simulink model "Disturbance_Rejection"  (R2025b)
settings: Solver=VariableStepAuto  StartTime=0.0  StopTime=t_sim  RelTol=1e-5  EnableMultiTasking=on
values from neighbouring files (symbols this model uses):
  Am = [0 1; -wn_model^2 -2*zeta_model*wn_model]    [MRC_DistReject.m]    (also in MRC_Simulation.m; MRC_Simulation1.m; MRC_Simulation2.m)
  Ap = [0   1;  -wn^2   -2*zeta*wn]    [MRC_DistReject.m]    (also in MRC_Simulation.m; MRC_Simulation1.m; MRC_Simulation2.m)
  Bm = [0; 1]    [MRC_DistReject.m]    (also in MRC_Simulation.m; MRC_Simulation1.m; MRC_Simulation2.m)
  Bp = [0;  1]    [MRC_DistReject.m]    (also in MRC_Simulation.m; MRC_Simulation1.m; MRC_Simulation2.m)
  Cm = eye(2)    [MRC_DistReject.m]    (also in MRC_Simulation.m; MRC_Simulation1.m; MRC_Simulation2.m)
  Dm = [0;0]    [MRC_DistReject.m]    (also in MRC_Simulation.m; MRC_Simulation1.m; MRC_Simulation2.m)
  step1 = 0    [MRC_DistReject.m]    (also in MRC_Simulation.m = 0.2; MRC_Simulation1.m = 0.2; MRC_Simulation2.m = 0.2)
  step2 = 0    [MRC_DistReject.m]    (also in MRC_Simulation.m = -0.2; MRC_Simulation1.m = -0.2; MRC_Simulation2.m = -0.2)
  t_off = 0    [MRC_DistReject.m]    (also in MRC_Simulation.m = 5; MRC_Simulation1.m = 5; MRC_Simulation2.m = 5)
  t_on = 0    [MRC_DistReject.m]    (also in MRC_Simulation.m; MRC_Simulation1.m; MRC_Simulation2.m = 0.25)
undefined symbols (not defined in the file or in its folder): MRC_Effort
settings Model: Creator=Kelvin  LastModifiedBy=HP
settings SolverCC: AlgebraicLoopSolver=TrustRegion
settings DataIOCC: LimitDataPoints=on  SaveFormat=Array  SignalLoggingSaveFormat=ModelDataLogs  ReturnWorkspaceOutputs=off
settings OptimizationCC: ExpressionDepthLimit=2147483647.0  LifeSpan=inf
settings DebuggingCC: UnderspecifiedInitializationDetection=Classic  MergeDetectMultiDrivingBlocksExec=none  SolverPrmCheckMsg=warning  FcnCallInpInsideContextMsg=warning  UnconnectedInputMsg=warning  UnconnectedOutputMsg=warning  UnconnectedLineMsg=warning  StateNameClashWarn=warning  SFUnexpectedBacktrackingDiag=warning  SFNoUnconditionalDefaultTransitionDiag=warning  SFExecutionAtInitializationDiag=none  ArithmeticOperatorsInVariantConditions=warning
settings HardwareCC: ProdBitPerPointer=32.0  ProdBitPerSizeT=32.0  ProdBitPerPtrDiffT=32.0  ProdLargestAtomicFloat=None  ProdIntDivRoundTo=Undefined  ProdEndianess=Unspecified  ProdWordSize=32.0  ProdHWDeviceType=32-bit Generic
settings ModelReferenceCC: PropagateSignalLabelsOutOfModel=off
settings SFSimCC: SimUseLocalCustomCode=off  CustomCodeUndefinedFunction=UseInterfaceOnly
settings RTWCC: RTWUseLocalCustomCode=off  GPUComputeCapability=3.5
settings CodeAppCC: StateflowObjectComments=on
settings GRTTargetCC: TargetLangStandard=C89/C90 (ANSI)  CombineOutputUpdateFcns=off  GRTInterface=on
settings ConfigComp: CovMetricSettings=dw  CovSaveCumulativeToWorkspaceVar=on  CovSaveSingleToWorkspaceVar=on  CovExternalEMLEnable=off

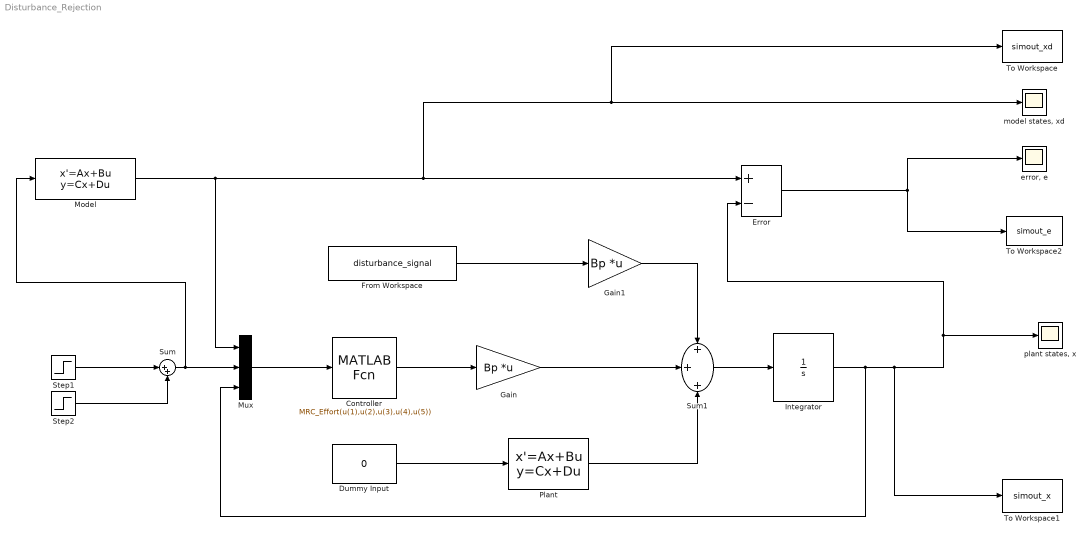
== system Disturbance_Rejection ==
  Controller : MATLABFcn  MATLABFcn=MRC_Effort(u(1),u(2),u(3),u(4),u(5))
  Dummy Input : Constant  Value=0
  Error : Sum  Inputs=+-
  From Workspace : FromWorkspace  VariableName=disturbance_signal
  Gain : Gain  Gain=Bp  Multiplication=Matrix(K*u)
  Gain1 : Gain  Gain=Bp  Multiplication=Matrix(K*u)
  Integrator : Integrator
  Model : StateSpace  A=Am  B=Bm  C=Cm  D=Dm  InitialCondition=0
  Mux : Mux  Inputs=3
  Plant : StateSpace  A=Ap  B=[0;0]  C=eye(2)  D=[0; 0]  InitialCondition=0
  Step1 : Step  Time=t_on  After=step1  SampleTime=0  ZeroCross=off
  Step2 : Step  Time=t_off  After=step2  SampleTime=0  ZeroCross=off
  Sum : Sum  Inputs=|++
  Sum1 : Sum  Inputs=+++
  To Workspace : ToWorkspace  VariableName=simout_xd  SaveFormat=Timeseries  SampleTime=-1
  To Workspace1 : ToWorkspace  VariableName=simout_x  SaveFormat=Timeseries  SampleTime=-1
  To Workspace2 : ToWorkspace  VariableName=simout_e  SaveFormat=Timeseries  SampleTime=-1
  "error, e" : Scope
      settings: ActiveDisplayYMinimum=-1  ActiveDisplayYMaximum=1  DataLoggingVariableName=ScopeData2
  "model states, xd" : Scope
      settings: TimeSpan=10  ActiveDisplayYMinimum=-1  ActiveDisplayYMaximum=1
  "plant states, x" : Scope
      settings: TimeSpan=10  ActiveDisplayYMinimum=-1.254638794084187  ActiveDisplayYMaximum=1.0606112059158137
  wires:
  Sum/1 -> Mux/2, Model/1
  Mux/1 -> Controller/1
  Model/1 -> Mux/1, Error/1, To Workspace/1, "model states, xd"/1
  Error/1 -> "error, e"/1, To Workspace2/1
  Step1/1 -> Sum/1
  Step2/1 -> Sum/2
  Dummy Input/1 -> Plant/1
  Plant/1 -> Sum1/3
  Controller/1 -> Gain/1
  From Workspace/1 -> Gain1/1
  Gain1/1 -> Sum1/1
  Gain/1 -> Sum1/2
  Sum1/1 -> Integrator/1
  Integrator/1 -> Mux/3, To Workspace1/1, Error/2, "plant states, x"/1
